simulink model "Hall"  (R2024a)
settings: Solver=FixedStepAuto  StartTime=0.0  StopTime=inf  FixedStep=1e-6  RelTol=1e-3
model workspace (MAT data in the model file):
  IntegraionGain = 1
undefined symbols (not defined in the file): DiscIntNeverNeededParam
libraries: simulink x20, simulink_extras x2
settings Model: Creator=wsl  LastModifiedBy=wsl

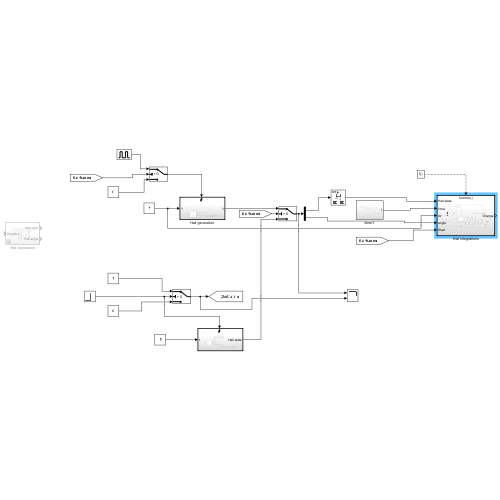
[thumbnail: Simulink's stored preview of the top-level diagram]
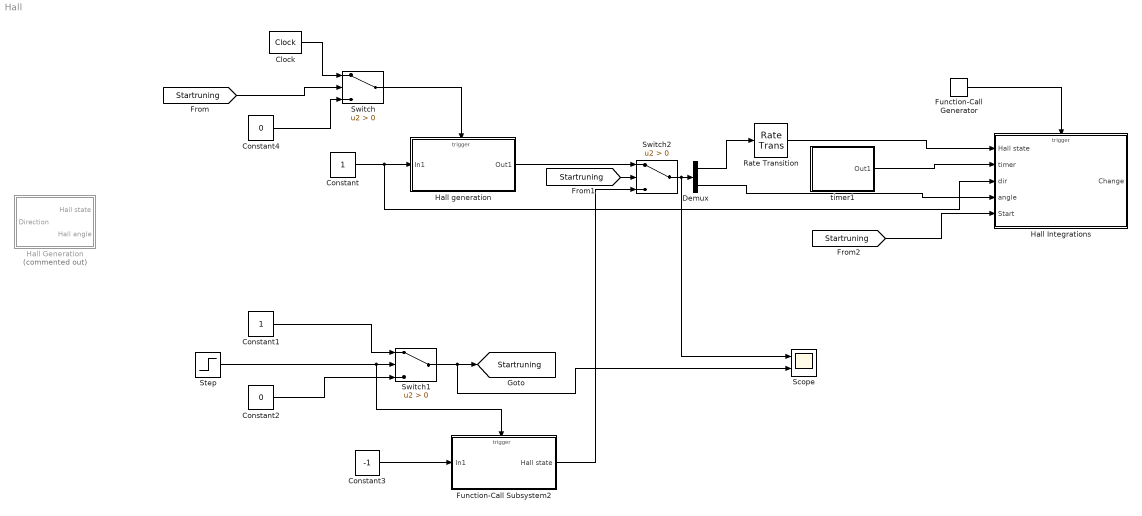
== system Hall ==
  Clock : simulink_extras/Flip Flops/Clock  period=0.02
  Constant : Constant
  Constant1 : Constant
  Constant2 : Constant  Value=0
  Constant3 : Constant  Value=-1
  Constant4 : Constant  Value=0
  Demux : Demux  Outputs=2
  Function-Call Generator : simulink/Ports & Subsystems/Function-Call Generator  sample_time=0.0001  numberOfIterations=1  DisallowWideOutput=off
  Function-Call Subsystem2 : Subsystem  TreatAsAtomicUnit=on
  Hall Generation : Subsystem  Commented=on
  Hall Integrations : Subsystem  TreatAsAtomicUnit=on
  Hall generation : Subsystem  TreatAsAtomicUnit=on
  Rate Transition : RateTransition  Integrity=off
  Scope : Scope  NumInputPorts=2
  Step : Step  Time=0.01
  Switch : Switch  Criteria=u2 > Threshold  SaturateOnIntegerOverflow=off  InputSameDT=off
  Switch1 : Switch  Criteria=u2 > Threshold  SaturateOnIntegerOverflow=off  InputSameDT=off
  Switch2 : Switch  Criteria=u2 > Threshold  SaturateOnIntegerOverflow=off  InputSameDT=off
  timer1 : Subsystem
  tag scope: Startruning=global
  wires:
  Function-Call Generator/1 -> Hall Integrations/Trigger
  Rate Transition/1 -> Hall Integrations/1(Hall state)
  Constant/1 -> Hall Integrations/3(dir), Hall generation/1(In1)
  timer1/1(Out1) -> Hall Integrations/2(timer)
  Switch/1 -> Hall generation/Trigger
  Clock/1 -> Switch/1
  Step/1 -> Function-Call Subsystem2/Trigger, Switch1/2
  Switch1/1 -> Scope/2, [Startruning]
  Constant1/1 -> Switch1/1
  Constant2/1 -> Switch1/3
  [Startruning] -> Switch/2
  Constant3/1 -> Function-Call Subsystem2/1(In1)
  [Startruning] -> Switch2/2
  Function-Call Subsystem2/1(Hall state) -> Switch2/3
  Hall generation/1(Out1) -> Switch2/1
  Switch2/1 -> Scope/1, Demux/1
  Demux/1 -> Rate Transition/1
  Demux/2 -> Hall Integrations/4(angle)
  Constant4/1 -> Switch/3
  [Startruning] -> Hall Integrations/5(Start)

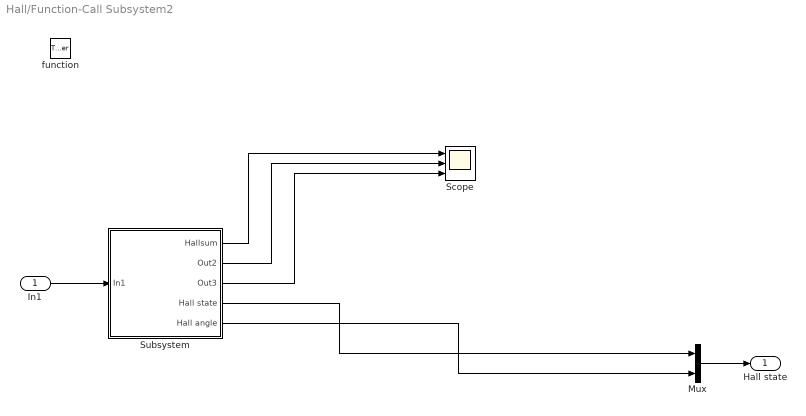
== system Hall/Function-Call Subsystem2 ==
  In1 : Inport
  function : TriggerPort  VariantControl=(inherit)
  Mux : Mux  Inputs=2
  Scope : Scope  NumInputPorts=3
  Subsystem : Subsystem
  Hall state : Outport
  wires:
  In1/1 -> Subsystem/1(In1)
  Subsystem/1(Hallsum) -> Scope/1
  Subsystem/2(Out2) -> Scope/2
  Subsystem/3(Out3) -> Scope/3
  Subsystem/5(Hall angle) -> Mux/2
  Mux/1 -> Hall state/1
  Subsystem/4(Hall state) -> Mux/1

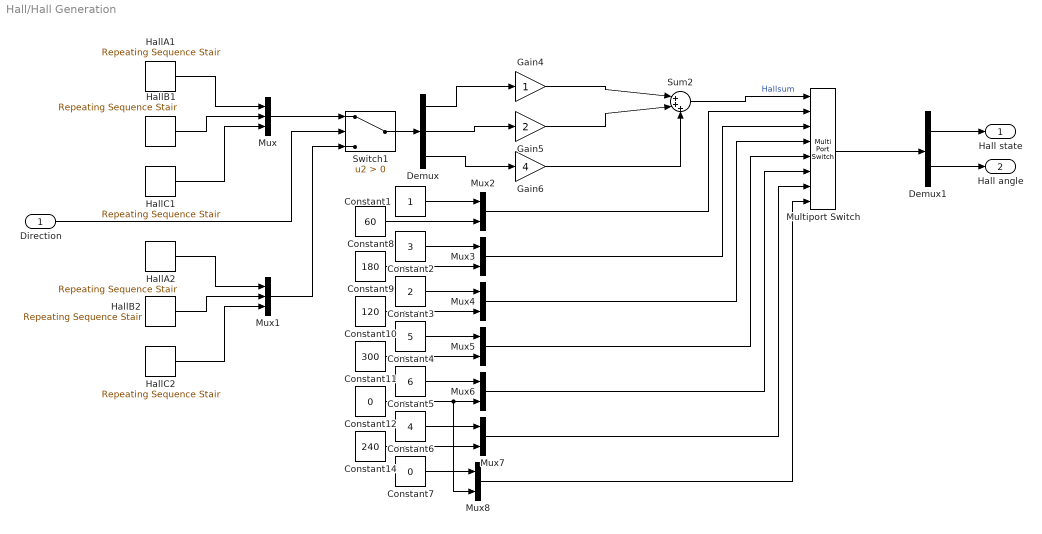
== system Hall/Hall Generation ==
  Direction : Inport
  Constant1 : Constant
  Constant10 : Constant  Value=120
  Constant11 : Constant  Value=300
  Constant12 : Constant  Value=0
  Constant14 : Constant  Value=240
  Constant2 : Constant  Value=3
  Constant3 : Constant  Value=2
  Constant4 : Constant  Value=5
  Constant5 : Constant  Value=6
  Constant6 : Constant  Value=4
  Constant7 : Constant  Value=0
  Constant8 : Constant  Value=60
  Constant9 : Constant  Value=180
  Demux : Demux  Outputs=3
  Demux1 : Demux  Outputs=2
  Gain4 : Gain
  Gain5 : Gain  Gain=2
  Gain6 : Gain  Gain=4
  HallA1 : simulink/Sources/Repeating Sequence Stair  OutValues=[1 1 1 1 0 0 0 0 0 0 1 1]'  tsamp=-1  OutMin=[]  OutMax=[]  OutDataTypeStr=double  OutputDataTypeScalingMode=double  OutDataType=fixdt(0,8)  ConRadixGroup=Best Precision: Vector-wise  OutScaling=2^-12
  HallA2 : simulink/Sources/Repeating Sequence Stair  OutValues=[1 0 0 0 1 1]'  tsamp=-1  OutMin=[]  OutMax=[]  OutDataTypeStr=double  OutputDataTypeScalingMode=double  OutDataType=fixdt(0,8)  ConRadixGroup=Best Precision: Vector-wise  OutScaling=2^-12
  HallB1 : simulink/Sources/Repeating Sequence Stair  OutValues=[0 0 1 1 1 1 1 1 0 0 0 0]'  tsamp=-1  OutMin=[]  OutMax=[]  OutDataTypeStr=double  OutputDataTypeScalingMode=double  OutDataType=fixdt(0,8)  ConRadixGroup=Best Precision: Vector-wise  OutScaling=2^-12
  HallB2 : simulink/Sources/Repeating Sequence Stair  OutValues=[0 0 1 1 1 0]'  tsamp=-1  OutMin=[]  OutMax=[]  OutDataTypeStr=double  OutputDataTypeScalingMode=double  OutDataType=fixdt(0,8)  ConRadixGroup=Best Precision: Vector-wise  OutScaling=2^-12
  HallC1 : simulink/Sources/Repeating Sequence Stair  OutValues=[0 0 0 0 0 0 1 1 1 1 1 1]'  tsamp=-1  OutMin=[]  OutMax=[]  OutDataTypeStr=double  OutputDataTypeScalingMode=double  OutDataType=fixdt(0,8)  ConRadixGroup=Best Precision: Vector-wise  OutScaling=2^-12
  HallC2 : simulink/Sources/Repeating Sequence Stair  OutValues=[1 1 1 0 0 0 ]'  tsamp=-1  OutMin=[]  OutMax=[]  OutDataTypeStr=double  OutputDataTypeScalingMode=double  OutDataType=fixdt(0,8)  ConRadixGroup=Best Precision: Vector-wise  OutScaling=2^-12
  Multiport Switch : MultiPortSwitch  Inputs=6  DataPortForDefault=Additional data port  SaturateOnIntegerOverflow=off  InputSameDT=off
  Mux : Mux  Inputs=3
  Mux1 : Mux  Inputs=3
  Mux{2..8} (7 alike) : Mux  Inputs=2
  Sum2 : Sum  Inputs=|+++
  Switch1 : Switch  Criteria=u2 > Threshold  SaturateOnIntegerOverflow=off  InputSameDT=off
  Hall state : Outport
  Hall angle : Outport  Port=2
  wires:
  HallC2/1 -> Mux1/3
  Mux/1 -> Switch1/1
  Demux/2 -> Gain5/1
  Gain5/1 -> Sum2/2
  Gain4/1 -> Sum2/1
  Gain6/1 -> Sum2/3
  HallA1/1 -> Mux/1
  HallB1/1 -> Mux/2
  Demux/3 -> Gain6/1
  Demux/1 -> Gain4/1
  Switch1/1 -> Demux/1
  HallA2/1 -> Mux1/1
  HallB2/1 -> Mux1/2
  Mux1/1 -> Switch1/3
  HallC1/1 -> Mux/3
  Sum2/1 -> Multiport Switch/1  "Hallsum"
  Direction/1 -> Switch1/2
  Constant1/1 -> Mux2/1
  Constant8/1 -> Mux2/2
  Mux2/1 -> Multiport Switch/2
  Constant9/1 -> Mux3/2
  Constant2/1 -> Mux3/1
  Mux3/1 -> Multiport Switch/3
  Constant3/1 -> Mux4/1
  Constant10/1 -> Mux4/2
  Mux4/1 -> Multiport Switch/4
  Constant4/1 -> Mux5/1
  Constant11/1 -> Mux5/2
  Mux5/1 -> Multiport Switch/5
  Constant5/1 -> Mux6/1
  Constant12/1 -> Mux8/2, Mux6/2
  Mux6/1 -> Multiport Switch/6
  Constant6/1 -> Mux7/1
  Constant14/1 -> Mux7/2
  Mux7/1 -> Multiport Switch/7
  Constant7/1 -> Mux8/1
  Mux8/1 -> Multiport Switch/8
  Multiport Switch/1 -> Demux1/1
  Demux1/1 -> Hall state/1
  Demux1/2 -> Hall angle/1

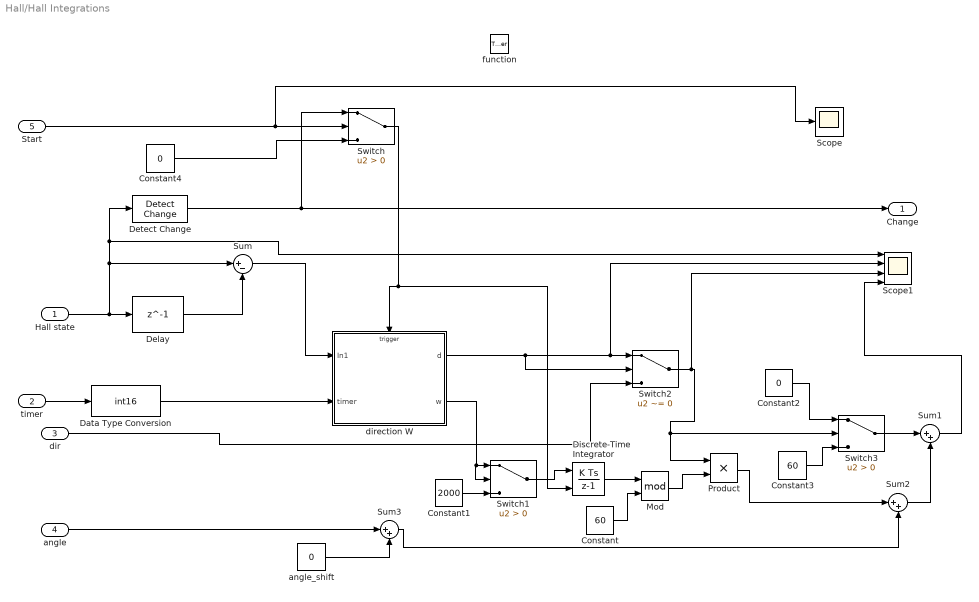
== system Hall/Hall Integrations ==
  Hall state : Inport
  timer : Inport  Port=2
  dir : Inport  Port=3
  angle : Inport  Port=4
  Start : Inport  Port=5
  function : TriggerPort  TriggerType=function-call  VariantControl=(inherit)
  Constant : Constant  Value=60
  Constant1 : Constant  Value=2000
  Constant2 : Constant  Value=0
  Constant3 : Constant  Value=60
  Constant4 : Constant  Value=0
  Data Type Conversion : DataTypeConversion  OutDataTypeStr=int16  ConvertRealWorld=Stored Integer (SI)  SaturateOnIntegerOverflow=off  RndMeth=Floor
  Delay : Delay  DelayLength=1  InitialCondition=0
  Detect Change : simulink/Logic and Bit Operations/Detect Change  vinit=0  OutDataTypeStr=boolean
  Discrete-Time Integrator : DiscreteIntegrator  ExternalReset=rising  SampleTime=-1  ICPrevOutput=DiscIntNeverNeededParam  ICPrevScaledInput=DiscIntNeverNeededParam
  Mod : Math  Operator=mod
  Product : Product
  Scope : Scope
  Scope1 : Scope  NumInputPorts=4
  Sum : Sum  Inputs=|+-
  Sum1 : Sum  Inputs=|++
  Sum2 : Sum  Inputs=|++
  Sum3 : Sum  Inputs=|++
  Switch : Switch  Criteria=u2 > Threshold  SaturateOnIntegerOverflow=off  InputSameDT=off
  Switch1 : Switch  Criteria=u2 > Threshold  SaturateOnIntegerOverflow=off  InputSameDT=off
  Switch2 : Switch  Criteria=u2 ~= 0  SaturateOnIntegerOverflow=off  InputSameDT=off
  Switch3 : Switch  Criteria=u2 > Threshold  SaturateOnIntegerOverflow=off  InputSameDT=off
  angle_shift : Constant  Value=0
  direction W : Subsystem  TreatAsAtomicUnit=on
  Change : Outport
  wires:
  Hall state/1 -> Delay/1, Sum/1, Scope1/1, Detect Change/1
  Detect Change/1 -> Switch/1, Change/1
  Delay/1 -> Sum/2
  Sum/1 -> direction W/1(In1)
  timer/1 -> Data Type Conversion/1
  Data Type Conversion/1 -> direction W/2(timer)
  Constant1/1 -> Switch1/3
  direction W/2(w) -> Switch1/2, Switch1/1
  Switch1/1 -> Discrete-Time Integrator/1
  dir/1 -> Switch2/3
  Switch2/1 -> Scope1/3, Product/1, Switch3/2
  direction W/1(d) -> Scope1/2, Switch2/1, Switch2/2
  Product/1 -> Sum2/1
  Constant2/1 -> Switch3/1
  Constant3/1 -> Switch3/3
  Switch3/1 -> Sum1/1
  Sum2/1 -> Sum1/2
  angle/1 -> Sum3/1
  Sum3/1 -> Sum2/2
  angle_shift/1 -> Sum3/2
  Start/1 -> Scope/1, Switch/2
  Switch/1 -> Discrete-Time Integrator/2, direction W/Trigger
  Constant4/1 -> Switch/3
  Sum1/1 -> Scope1/4
  Discrete-Time Integrator/1 -> Mod/1
  Mod/1 -> Product/2
  Constant/1 -> Mod/2

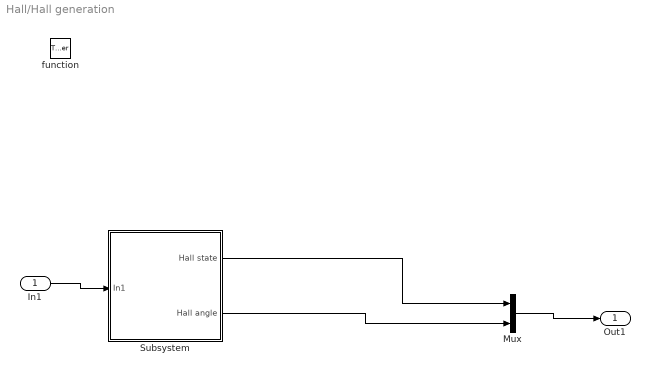
== system Hall/Hall generation ==
  In1 : Inport
  function : TriggerPort  VariantControl=(inherit)
  Mux : Mux  Inputs=2
  Subsystem : Subsystem
  Out1 : Outport
  wires:
  In1/1 -> Subsystem/1(In1)
  Subsystem/1(Hall state) -> Mux/1
  Subsystem/2(Hall angle) -> Mux/2
  Mux/1 -> Out1/1

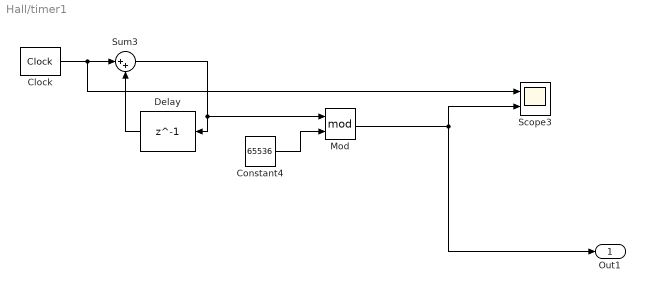
== system Hall/timer1 ==
  Clock : simulink_extras/Flip Flops/Clock  period=5e-5
  Constant4 : Constant  Value=65536
  Delay : Delay  DelayLength=1  InitialCondition=0  UseCircularBuffer=on
  Mod : Math  Operator=mod
  Scope3 : Scope  NumInputPorts=2
  Sum3 : Sum  Inputs=|++
  Out1 : Outport
  wires:
  Delay/1 -> Sum3/2
  Constant4/1 -> Mod/2
  Clock/1 -> Scope3/1, Sum3/1
  Mod/1 -> Out1/1, Scope3/2
  Sum3/1 -> Mod/1, Delay/1

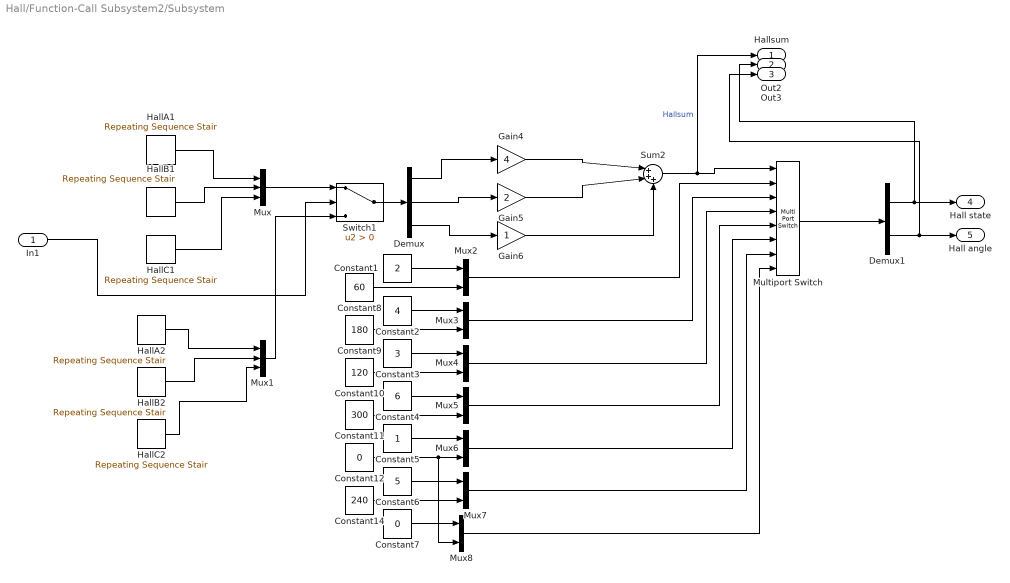
== system Hall/Function-Call Subsystem2/Subsystem ==
  In1 : Inport
  Constant1 : Constant  Value=2
  Constant10 : Constant  Value=120
  Constant11 : Constant  Value=300
  Constant12 : Constant  Value=0
  Constant14 : Constant  Value=240
  Constant2 : Constant  Value=4
  Constant3 : Constant  Value=3
  Constant4 : Constant  Value=6
  Constant5 : Constant
  Constant6 : Constant  Value=5
  Constant7 : Constant  Value=0
  Constant8 : Constant  Value=60
  Constant9 : Constant  Value=180
  Demux : Demux  Outputs=3
  Demux1 : Demux  Outputs=2
  Gain4 : Gain  Gain=4
  Gain5 : Gain  Gain=2
  Gain6 : Gain
  HallA1 : simulink/Sources/Repeating Sequence Stair  OutValues=[1 1 0 0 0 1]'  tsamp=-1  OutMin=[]  OutMax=[]  OutDataTypeStr=double  OutputDataTypeScalingMode=double  OutDataType=fixdt(0,8)  ConRadixGroup=Best Precision: Vector-wise  OutScaling=2^-12
  HallA2 : simulink/Sources/Repeating Sequence Stair  OutValues=[1 1 0 0 0 1]'  tsamp=-1  OutMin=[]  OutMax=[]  OutDataTypeStr=double  OutputDataTypeScalingMode=double  OutDataType=fixdt(0,8)  ConRadixGroup=Best Precision: Vector-wise  OutScaling=2^-12
  HallB1 : simulink/Sources/Repeating Sequence Stair  OutValues=[ 0 0 0 1 1 1]'  tsamp=-1  OutMin=[]  OutMax=[]  OutDataTypeStr=double  OutputDataTypeScalingMode=double  OutDataType=fixdt(0,8)  ConRadixGroup=Best Precision: Vector-wise  OutScaling=2^-12
  HallB2 : simulink/Sources/Repeating Sequence Stair  OutValues=[0 1 1 1 0 0 ]'  tsamp=-1  OutMin=[]  OutMax=[]  OutDataTypeStr=double  OutputDataTypeScalingMode=double  OutDataType=fixdt(0,8)  ConRadixGroup=Best Precision: Vector-wise  OutScaling=2^-12
  HallC1 : simulink/Sources/Repeating Sequence Stair  OutValues=[ 0 1 1 1 0 0]'  tsamp=-1  OutMin=[]  OutMax=[]  OutDataTypeStr=double  OutputDataTypeScalingMode=double  OutDataType=fixdt(0,8)  ConRadixGroup=Best Precision: Vector-wise  OutScaling=2^-12
  HallC2 : simulink/Sources/Repeating Sequence Stair  OutValues=[0 0 0 1 1 1 ]'  tsamp=-1  OutMin=[]  OutMax=[]  OutDataTypeStr=double  OutputDataTypeScalingMode=double  OutDataType=fixdt(0,8)  ConRadixGroup=Best Precision: Vector-wise  OutScaling=2^-12
  Multiport Switch : MultiPortSwitch  Inputs=6  DataPortForDefault=Additional data port  SaturateOnIntegerOverflow=off  InputSameDT=off
  Mux : Mux  Inputs=3
  Mux1 : Mux  Inputs=3
  Mux{2..8} (7 alike) : Mux  Inputs=2
  Sum2 : Sum  Inputs=|+++
  Switch1 : Switch  Criteria=u2 > Threshold  SaturateOnIntegerOverflow=off  InputSameDT=off
  Hallsum : Outport
  Out2 : Outport  Port=2
  Out3 : Outport  Port=3
  Hall state : Outport  Port=4
  Hall angle : Outport  Port=5
  wires:
  Constant3/1 -> Mux4/1
  Mux3/1 -> Multiport Switch/3
  Gain5/1 -> Sum2/2
  Constant12/1 -> Mux8/2, Mux6/2
  Demux/1 -> Gain4/1
  Constant10/1 -> Mux4/2
  Constant7/1 -> Mux8/1
  Mux6/1 -> Multiport Switch/6
  Mux8/1 -> Multiport Switch/8
  Multiport Switch/1 -> Demux1/1
  Mux5/1 -> Multiport Switch/5
  Gain6/1 -> Sum2/3
  Demux1/2 -> Hall angle/1, Out3/1
  Mux7/1 -> Multiport Switch/7
  Constant8/1 -> Mux2/2
  Mux2/1 -> Multiport Switch/2
  Constant6/1 -> Mux7/1
  Sum2/1 -> Hallsum/1, Multiport Switch/1  "Hallsum"
  Gain4/1 -> Sum2/1
  Mux4/1 -> Multiport Switch/4
  Constant2/1 -> Mux3/1
  HallB1/1 -> Mux/2
  Constant1/1 -> Mux2/1
  HallB2/1 -> Mux1/2
  HallC2/1 -> Mux1/3
  HallA1/1 -> Mux/1
  Constant9/1 -> Mux3/2
  Constant14/1 -> Mux7/2
  HallC1/1 -> Mux/3
  Demux/3 -> Gain6/1
  Constant4/1 -> Mux5/1
  Constant5/1 -> Mux6/1
  Demux1/1 -> Hall state/1, Out2/1
  Switch1/1 -> Demux/1
  HallA2/1 -> Mux1/1
  Mux/1 -> Switch1/1
  Constant11/1 -> Mux5/2
  Mux1/1 -> Switch1/3
  In1/1 -> Switch1/2
  Demux/2 -> Gain5/1

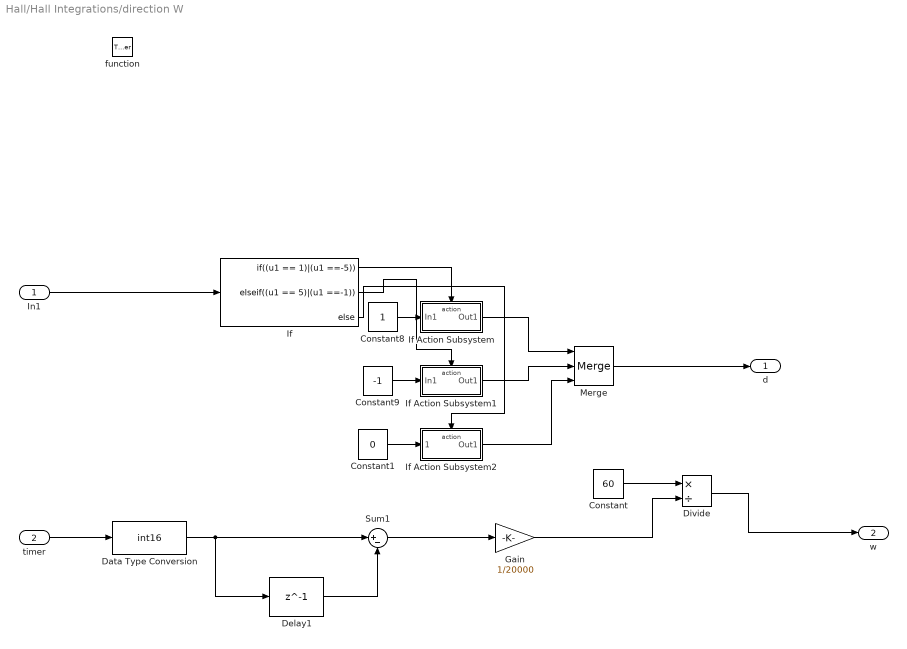
== system Hall/Hall Integrations/direction W ==
  In1 : Inport
  timer : Inport  Port=2
  function : TriggerPort  VariantControl=(inherit)
  Constant : Constant  Value=60
  Constant1 : Constant  Value=0
  Constant8 : Constant
  Constant9 : Constant  Value=-1
  Data Type Conversion : DataTypeConversion  OutDataTypeStr=int16  ConvertRealWorld=Stored Integer (SI)  SaturateOnIntegerOverflow=off  RndMeth=Floor
  Delay1 : Delay  DelayLength=1  InitialCondition=0
  Divide : Product  Inputs=*/
  Gain : Gain  Gain=1/20000
  If : If  IfExpression=(u1 == 1)|(u1 ==-5)  ElseIfExpressions=(u1 == 5)|(u1 ==-1)
  If Action Subsystem : Subsystem  TreatAsAtomicUnit=on
  If Action Subsystem1 : Subsystem  TreatAsAtomicUnit=on
  If Action Subsystem2 : Subsystem  TreatAsAtomicUnit=on
  Merge : Merge  Inputs=3
  Sum1 : Sum  Inputs=|+-
  d : Outport
  w : Outport  Port=2
  wires:
  If Action Subsystem1/1(Out1) -> Merge/2
  Constant8/1 -> If Action Subsystem/1(In1)
  If/2 -> If Action Subsystem1/Action
  If/1 -> If Action Subsystem/Action
  If Action Subsystem2/1(Out1) -> Merge/3
  If/3 -> If Action Subsystem2/Action
  Constant9/1 -> If Action Subsystem1/1(In1)
  If Action Subsystem/1(Out1) -> Merge/1
  In1/1 -> If/1
  Merge/1 -> d/1
  Sum1/1 -> Gain/1
  Data Type Conversion/1 -> Delay1/1, Sum1/1
  Delay1/1 -> Sum1/2
  timer/1 -> Data Type Conversion/1
  Constant/1 -> Divide/1
  Divide/1 -> w/1
  Gain/1 -> Divide/2
  Constant1/1 -> If Action Subsystem2/1(derection)

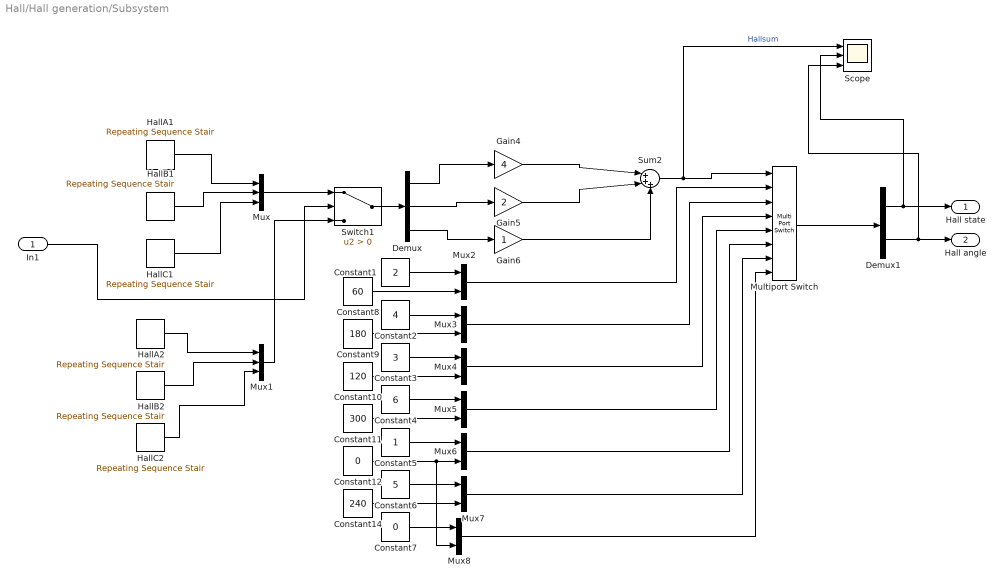
== system Hall/Hall generation/Subsystem ==
  In1 : Inport
  Constant1 : Constant  Value=2
  Constant10 : Constant  Value=120
  Constant11 : Constant  Value=300
  Constant12 : Constant  Value=0
  Constant14 : Constant  Value=240
  Constant2 : Constant  Value=4
  Constant3 : Constant  Value=3
  Constant4 : Constant  Value=6
  Constant5 : Constant
  Constant6 : Constant  Value=5
  Constant7 : Constant  Value=0
  Constant8 : Constant  Value=60
  Constant9 : Constant  Value=180
  Demux : Demux  Outputs=3
  Demux1 : Demux  Outputs=2
  Gain4 : Gain  Gain=4
  Gain5 : Gain  Gain=2
  Gain6 : Gain
  HallA1 : simulink/Sources/Repeating Sequence Stair  OutValues=[1 1 0 0 0 1]'  tsamp=-1  OutMin=[]  OutMax=[]  OutDataTypeStr=double  OutputDataTypeScalingMode=double  OutDataType=fixdt(0,8)  ConRadixGroup=Best Precision: Vector-wise  OutScaling=2^-12
  HallA2 : simulink/Sources/Repeating Sequence Stair  OutValues=[1 1 0 0 0 1]'  tsamp=-1  OutMin=[]  OutMax=[]  OutDataTypeStr=double  OutputDataTypeScalingMode=double  OutDataType=fixdt(0,8)  ConRadixGroup=Best Precision: Vector-wise  OutScaling=2^-12
  HallB1 : simulink/Sources/Repeating Sequence Stair  OutValues=[ 0 0 0 1 1 1]'  tsamp=-1  OutMin=[]  OutMax=[]  OutDataTypeStr=double  OutputDataTypeScalingMode=double  OutDataType=fixdt(0,8)  ConRadixGroup=Best Precision: Vector-wise  OutScaling=2^-12
  HallB2 : simulink/Sources/Repeating Sequence Stair  OutValues=[0 1 1 1 0 0 ]'  tsamp=-1  OutMin=[]  OutMax=[]  OutDataTypeStr=double  OutputDataTypeScalingMode=double  OutDataType=fixdt(0,8)  ConRadixGroup=Best Precision: Vector-wise  OutScaling=2^-12
  HallC1 : simulink/Sources/Repeating Sequence Stair  OutValues=[ 0 1 1 1 0 0]'  tsamp=-1  OutMin=[]  OutMax=[]  OutDataTypeStr=double  OutputDataTypeScalingMode=double  OutDataType=fixdt(0,8)  ConRadixGroup=Best Precision: Vector-wise  OutScaling=2^-12
  HallC2 : simulink/Sources/Repeating Sequence Stair  OutValues=[0 0 0 1 1 1 ]'  tsamp=-1  OutMin=[]  OutMax=[]  OutDataTypeStr=double  OutputDataTypeScalingMode=double  OutDataType=fixdt(0,8)  ConRadixGroup=Best Precision: Vector-wise  OutScaling=2^-12
  Multiport Switch : MultiPortSwitch  Inputs=6  DataPortForDefault=Additional data port  SaturateOnIntegerOverflow=off  InputSameDT=off
  Mux : Mux  Inputs=3
  Mux1 : Mux  Inputs=3
  Mux{2..8} (7 alike) : Mux  Inputs=2
  Scope : Scope  NumInputPorts=3
  Sum2 : Sum  Inputs=|+++
  Switch1 : Switch  Criteria=u2 > Threshold  SaturateOnIntegerOverflow=off  InputSameDT=off
  Hall state : Outport
  Hall angle : Outport  Port=2
  wires:
  Constant3/1 -> Mux4/1
  Mux3/1 -> Multiport Switch/3
  Gain5/1 -> Sum2/2
  Constant12/1 -> Mux8/2, Mux6/2
  Demux/1 -> Gain4/1
  Constant10/1 -> Mux4/2
  Constant7/1 -> Mux8/1
  Mux6/1 -> Multiport Switch/6
  Mux8/1 -> Multiport Switch/8
  Multiport Switch/1 -> Demux1/1
  Mux5/1 -> Multiport Switch/5
  Gain6/1 -> Sum2/3
  Demux1/2 -> Scope/3, Hall angle/1
  Mux7/1 -> Multiport Switch/7
  Constant8/1 -> Mux2/2
  Mux2/1 -> Multiport Switch/2
  Constant6/1 -> Mux7/1
  Sum2/1 -> Scope/1, Multiport Switch/1  "Hallsum"
  Gain4/1 -> Sum2/1
  Mux4/1 -> Multiport Switch/4
  Constant2/1 -> Mux3/1
  HallB1/1 -> Mux/2
  Constant1/1 -> Mux2/1
  HallB2/1 -> Mux1/2
  HallC2/1 -> Mux1/3
  HallA1/1 -> Mux/1
  Constant9/1 -> Mux3/2
  Constant14/1 -> Mux7/2
  HallC1/1 -> Mux/3
  Demux/3 -> Gain6/1
  Constant4/1 -> Mux5/1
  Constant5/1 -> Mux6/1
  Switch1/1 -> Demux/1
  HallA2/1 -> Mux1/1
  Mux/1 -> Switch1/1
  Constant11/1 -> Mux5/2
  Mux1/1 -> Switch1/3
  In1/1 -> Switch1/2
  Demux/2 -> Gain5/1
  Demux1/1 -> Scope/2, Hall state/1

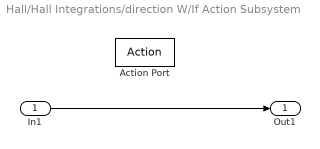
== system Hall/Hall Integrations/direction W/If Action Subsystem ==
  In1 : Inport
  Action Port : ActionPort  ActionPortLabel=if((u1 == 1)|(u1 ==-5))
  Out1 : Outport
  wires:
  In1/1 -> Out1/1

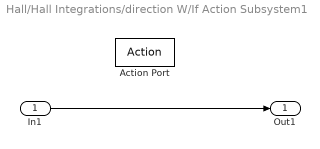
== system Hall/Hall Integrations/direction W/If Action Subsystem1 ==
  In1 : Inport
  Action Port : ActionPort  ActionPortLabel=elseif((u1 == 5)|(u1 ==-1))
  Out1 : Outport
  wires:
  In1/1 -> Out1/1

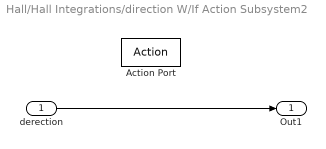
== system Hall/Hall Integrations/direction W/If Action Subsystem2 ==
  derection : Inport
  Action Port : ActionPort  ActionPortLabel=else
  Out1 : Outport
  wires:
  derection/1 -> Out1/1
